simulink model "Velocity_simulink_2019"  (R2024b)
settings: Solver=VariableStepAuto  StartTime=0.0  StopTime=10.0  RelTol=1e-3
libraries: simulink_extras x2, simulink x2
settings Model: Creator=Ashraf  LastModifiedBy=Abdulbaseer
settings SolverCC: AlgebraicLoopSolver=TrustRegion
settings DebuggingCC: UnconnectedInputMsg=warning  UnconnectedOutputMsg=warning  UnconnectedLineMsg=warning
settings ModelReferenceCC: EnableRefExpFcnMdlSchedulingChecks=on
settings SFSimCC: CustomCodeUndefinedFunction=UseInterfaceOnly
settings RTWCC: GPUComputeCapability=3.5

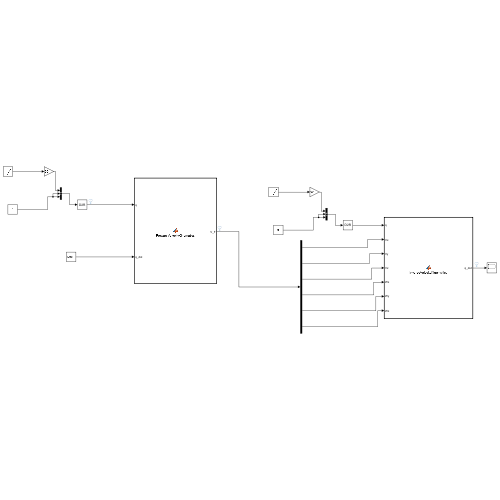
[thumbnail: Simulink's stored preview of the top-level diagram]
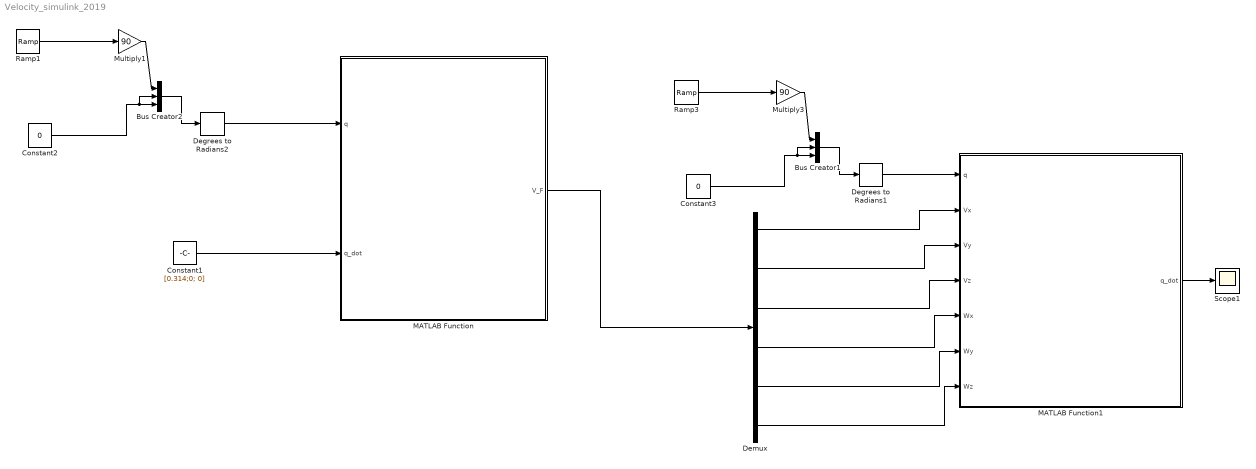
== system Velocity_simulink_2019 ==
  Bus Creator1 : BusCreator  Inputs=3
  Bus Creator2 : BusCreator  Inputs=3
  Constant1 : Constant  Value=[0.314;0; 0]
  Constant2 : Constant  Value=0
  Constant3 : Constant  Value=0
  Degrees to Radians1 : simulink_extras/Transformations/Degrees to Radians
  Degrees to Radians2 : simulink_extras/Transformations/Degrees to Radians
  Demux : Demux  Outputs=6
  MATLAB Function : MATLAB Function  TreatAsAtomicUnit=on
  MATLAB Function1 : MATLAB Function  TreatAsAtomicUnit=on
  Multiply1 : Gain  Gain=90
  Multiply3 : Gain  Gain=90
  Ramp1 : simulink/Sources/Ramp  slope=0.2  start=0  InitialOutput=0
  Ramp3 : simulink/Sources/Ramp  slope=0.2  start=0  InitialOutput=0
  Scope1 : Scope
  wires:
  Degrees to Radians1/1 -> MATLAB Function1/1(q)
  Multiply3/1 -> Bus Creator1/1
  Ramp3/1 -> Multiply3/1
  Constant3/1 -> Bus Creator1/2, Bus Creator1/3
  Bus Creator1/1 -> Degrees to Radians1/1
  MATLAB Function1/1(q_dot) -> Scope1/1
  Degrees to Radians2/1 -> MATLAB Function/1(q)
  Constant1/1 -> MATLAB Function/2(q_dot)
  MATLAB Function/1(V_F) -> Demux/1
  Demux/1 -> MATLAB Function1/2(Vx)
  Demux/2 -> MATLAB Function1/3(Vy)
  Demux/3 -> MATLAB Function1/4(Vz)
  Demux/4 -> MATLAB Function1/5(Wx)
  Demux/5 -> MATLAB Function1/6(Wy)
  Demux/6 -> MATLAB Function1/7(Wz)
  Ramp1/1 -> Multiply1/1
  Bus Creator2/1 -> Degrees to Radians2/1
  Constant2/1 -> Bus Creator2/2, Bus Creator2/3
  Multiply1/1 -> Bus Creator2/1

== matlab function Velocity_simulink_2019/MATLAB Function1 ==
  data: q input; q_dot output; Vx input; Vy input; Vz input; Wx input; Wy input; Wz input
function q_dot = InverseVelocityKinematics(q,Vx, Vy, Vz, Wx, Wy, Wz)
%#codegen
    % Define link lengths
    l0 = 0.097;   % Length of link 0
    l1 = 0.119;   % Length of link 1
    l2 = 0.119;   % Length of link 2
    pi=22/7;
    % Define DH parameters based on joint angles and link lengths
    DH_table = [q(1), l0, -0.014, pi/2;
                q(2), 0, l1, 0;
                q(3), 0, l2, 0];

    % Initialize transformation matrix and fixed-size Jacobian matrices
    T = eye(4);
    Jv = zeros(3, 3); % Pre-allocate 3x3 matrix for linear velocity Jacobian
    Jw = zeros(3, 3); % Pre-allocate 3x3 matrix for angular velocity Jacobian
    Z0 = [0;0;1];
    O0 = [0;0;0];
    Ot = zeros(3, 3);
    zt = zeros(3, 3);
    V_F = [Vx; Vy; Vz; Wx; Wy; Wz];
    q_dot = zeros(3, 1);

    % Compute transformations and Jacobian entries
    for i = 1:3
        % Extract DH parameters
        theta = DH_table(i, 1);
        d = DH_table(i, 2);
        a = DH_table(i, 3);
        alpha = DH_table(i, 4);

        % Transformation matrix for current joint
        Ti = [cos(theta), -sin(theta)*cos(alpha), sin(theta)*sin(alpha), a*cos(theta);
              sin(theta), cos(theta)*cos(alpha), -cos(theta)*sin(alpha), a*sin(theta);
              0, sin(alpha), cos(alpha), d;
              0, 0, 0, 1];

        T = T * Ti;  % Update cumulative transformation

        % Get current joint's origin and Z-axis in the base frame
        Oi = T(1:3, 4);
        Ot(1:3, i) = Oi;
        Zi = T(1:3, 3);
        zt(1:3, i) = Zi;
       
    end

    % Compute Jacobian columns
    Jv(:,1) = cross(Z0, Ot(1:3,3) - O0);  % Linear velocity component for revolute joint
    Jw(:, 1) = Z0;        % Assign to pre-allocated Jw
    for i=2:3
        Jv(:, i) = cross(zt(:,i-1), Ot(1:3,3) - Ot(1:3,i-1));     % Assign to pre-allocated Jv
        Jw(:, i) = zt(:,i-1);        % Assign to pre-allocated Jw
    end
    % Combine linear and angular velocity Jacobian parts
    J = [Jv; Jw];

    % Compute Moore-Penrose pseudo-inverse of the Jacobian for inverse kinematics
    J_inv = pinv(J);  % Direct pseudo-inverse to yield a 3x6 matrix

    % Calculate joint velocities from inverse velocity kinematics
    q_dot = (J_inv * V_F);

end

== matlab function Velocity_simulink_2019/MATLAB Function ==
  data: q input; V_F output; q_dot input
function V_F = ForwardVelocityKinematics(q, q_dot)
%#codegen
    % Define link lengths
    l0 = 0.097;   % Length of link 0
    l1 = 0.119;   % Length of link 1
    l2 = 0.119;   % Length of link 2
    pi=22/7;
    % Define DH parameters based on joint angles and link lengths
    DH_table = [q(1), l0, -0.014, pi/2;
                q(2), 0, l1, 0;
                q(3), 0, l2, 0];

    % Initialize transformation matrix and fixed-size Jacobian matrices
    T = eye(4);
    Jv = zeros(3, 3); % Pre-allocate 3x3 matrix for linear velocity Jacobian
    Jw = zeros(3, 3); % Pre-allocate 3x3 matrix for angular velocity Jacobian
    Z0 = [0;0;1];
    O0 = [0;0;0];
    Ot = zeros(3, 3);
    zt = zeros(3, 3);

    % Compute transformations and Jacobian entries
    for i = 1:3
        % Extract DH parameters
        theta = DH_table(i, 1);
        d = DH_table(i, 2);
        a = DH_table(i, 3);
        alpha = DH_table(i, 4);

        % Transformation matrix for current joint
        Ti = [cos(theta), -sin(theta)*cos(alpha), sin(theta)*sin(alpha), a*cos(theta);
              sin(theta), cos(theta)*cos(alpha), -cos(theta)*sin(alpha), a*sin(theta);
              0, sin(alpha), cos(alpha), d;
              0, 0, 0, 1];

        T = T * Ti;  % Update cumulative transformation

        % Get current joint's origin and Z-axis in the base frame
        Oi = T(1:3, 4);
        Ot(1:3, i) = Oi;
        Zi = T(1:3, 3);
        zt(1:3, i) = Zi;

       
    end

    % Compute Jacobian columns
    Jv(:,1) = cross(Z0, Ot(1:3,3) - O0);  % Linear velocity component for revolute joint
    Jw(:, 1) = Z0;        % Assign to pre-allocated Jw
    for i=2:3
        Jv(:, i) = cross(zt(:,i-1), Ot(1:3,3) - Ot(1:3,i-1));     % Assign to pre-allocated Jv
        Jw(:, i) = zt(:,i-1);        % Assign to pre-allocated Jw
    end
    % Combine linear and angular velocity Jacobian parts
    J = [Jv; Jw];

    % Compute forward velocity kinematics
    V_F = J * q_dot;
end
